simulink subsystem "celestialBodies"  (R2023b)
settings: Solver=VariableStepAuto  StartTime=0.0  StopTime=10.0  RelTol=1e-3
undefined symbols (not defined in the file or in its folder): Environment, phi, phi_dot, psi, psi_dot, theta, theta_dot
libraries: dyn_lib x2
settings Model: DataDictionary=Scenario.sldd  EnableAccessToBaseWorkspace=off  Creator=brent  LastModifiedBy=brent

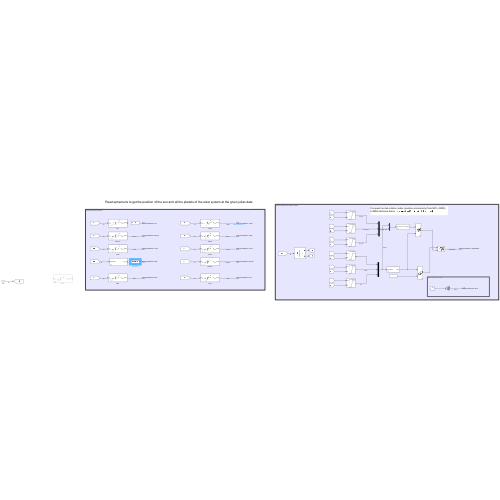
[thumbnail: Simulink's stored preview of the top-level diagram]
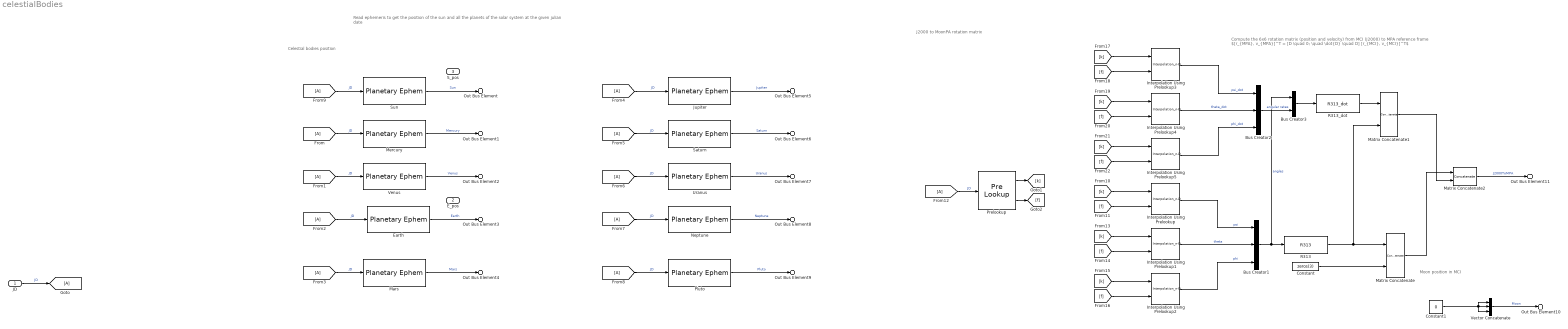
== system celestialBodies ==
  note: Compute the 6x6 rotation matrix (position and velocity) from MCI (J2000) to MPA reference frame $[r_{MPA}, v_{MPA}]^T = [D \quad 0; \quad \dot{D} \quad D] [r_{MCI}, v_{MCI}]^T$
  note: Read ephemeris to get the position of the sun and all the planets of the solar system at the given julian date
  note: Moon position in MCI
  note: J2000 to MoonPA rotation matrix
  note: Celestial bodies position
  JD : Inport
  E_pos : Inport  Port=2
  S_pos : Inport  Port=3
  Bus Creator1 : BusCreator  Inputs=psi,theta,phi
  Bus Creator2 : BusCreator  Inputs=psi_dot,theta_dot,phi_dot
  Bus Creator3 : BusCreator  Inputs=2
  Constant : Constant  Value=zeros(3)
  Constant1 : Constant  Value=0
  Earth : PlanetaryEphem  ephemerisModel=DE421  center=Moon  target=Earth  outputVelocity=off
  From{,1..9,12} (11 alike) : From
  Goto : Goto
  Interpolation Using Prelookup : Interpolation_n-D  NumberOfTableDimensions=1  Table=Environment.Moon.orientation.value(:,1)  InternalRulePriority=Speed
      settings: InputPortMap=u0,u1
  Interpolation Using Prelookup1 : Interpolation_n-D  NumberOfTableDimensions=1  Table=Environment.Moon.orientation.value(:,2)  InternalRulePriority=Speed
      settings: InputPortMap=u0,u1
  Interpolation Using Prelookup2 : Interpolation_n-D  NumberOfTableDimensions=1  Table=Environment.Moon.orientation.value(:,3)  InternalRulePriority=Speed
      settings: InputPortMap=u0,u1
  Interpolation Using Prelookup3 : Interpolation_n-D  NumberOfTableDimensions=1  Table=Environment.Moon.orientation_dot.value(:,1)  InternalRulePriority=Speed
      settings: InputPortMap=u0,u1
  Interpolation Using Prelookup4 : Interpolation_n-D  NumberOfTableDimensions=1  Table=Environment.Moon.orientation_dot.value(:,2)  InternalRulePriority=Speed
      settings: InputPortMap=u0,u1
  Interpolation Using Prelookup5 : Interpolation_n-D  NumberOfTableDimensions=1  Table=Environment.Moon.orientation_dot.value(:,3)  InternalRulePriority=Speed
      settings: InputPortMap=u0,u1
  Jupiter : PlanetaryEphem  ephemerisModel=DE421  center=Moon  target=Jupiter  outputVelocity=off
  Mars : PlanetaryEphem  ephemerisModel=DE421  center=Moon  target=Mars  outputVelocity=off
  Matrix Concatenate : Concatenate  Mode=Multidimensional array  ConcatenateDimension=2
  Matrix Concatenate1 : Concatenate  Mode=Multidimensional array  ConcatenateDimension=2
  Matrix Concatenate2 : Concatenate  Mode=Multidimensional array
  Mercury : PlanetaryEphem  ephemerisModel=DE421  center=Moon  target=Mercury  outputVelocity=off
  Neptune : PlanetaryEphem  ephemerisModel=DE421  center=Moon  target=Neptune  outputVelocity=off
  Pluto : PlanetaryEphem  ephemerisModel=DE421  center=Moon  target=Pluto  outputVelocity=off
  Prelookup : PreLookup  BreakpointsData=Environment.Moon.jd_interval.value  BeginIndexSearchUsingPreviousIndexResult=on  ExtrapMethod=Linear
  R313 : dyn_lib/R313
      settings: SourceProductName=Dynamics library
  R313_dot : dyn_lib/R313_dot
      settings: SourceProductName=Dynamics library
  Saturn : PlanetaryEphem  ephemerisModel=DE421  center=Moon  target=Saturn  outputVelocity=off
  "Sun " : PlanetaryEphem  ephemerisModel=DE421  center=Moon  target=Sun  outputVelocity=off
  Uranus : PlanetaryEphem  ephemerisModel=DE421  center=Moon  target=Uranus  outputVelocity=off
  Vector Concatenate : Concatenate  NumInputs=3
  Venus : PlanetaryEphem  ephemerisModel=DE421  center=Moon  target=Venus  outputVelocity=off
  Out Bus Element : Outport  PortName=celestialBodies  Element=Sun
  Out Bus Element1 : Outport  PortName=celestialBodies  Element=Mercury
  Out Bus Element2 : Outport  PortName=celestialBodies  Element=Venus
  Out Bus Element3 : Outport  PortName=celestialBodies  Element=Earth
  Out Bus Element4 : Outport  PortName=celestialBodies  Element=Mars
  Out Bus Element5 : Outport  PortName=celestialBodies  Element=Jupiter
  Out Bus Element6 : Outport  PortName=celestialBodies  Element=Saturn
  Out Bus Element7 : Outport  PortName=celestialBodies  Element=Uranus
  Out Bus Element8 : Outport  PortName=celestialBodies  Element=Neptune
  Out Bus Element9 : Outport  PortName=celestialBodies  Element=Pluto
  Out Bus Element10 : Outport  PortName=celestialBodies  Element=Moon
  Out Bus Element11 : Outport  PortName=celestialBodies  Element=J2000ToMPA
  wires:
  From/1 -> Mercury/1  "JD"
  From1/1 -> Venus/1  "JD"
  From3/1 -> Mars/1  "JD"
  From6/1 -> Uranus/1  "JD"
  From4/1 -> Jupiter/1  "JD"
  From5/1 -> Saturn/1  "JD"
  From7/1 -> Neptune/1  "JD"
  From8/1 -> Pluto/1  "JD"
  From9/1 -> "Sun "/1  "JD"
  Mercury/1 -> Out Bus Element1/1  "Mercury"
  Venus/1 -> Out Bus Element2/1  "Venus"
  Mars/1 -> Out Bus Element4/1  "Mars"
  Jupiter/1 -> Out Bus Element5/1  "Jupiter"
  Saturn/1 -> Out Bus Element6/1  "Saturn"
  Uranus/1 -> Out Bus Element7/1  "Uranus"
  Neptune/1 -> Out Bus Element8/1  "Neptune"
  Pluto/1 -> Out Bus Element9/1  "Pluto"
  JD/1 -> Goto/1  "JD"
  Prelookup/1 -> [k]
  Prelookup/2 -> [f]
  From12/1 -> Prelookup/1  "JD"
  [k] -> Interpolation Using Prelookup/1
  [f] -> Interpolation Using Prelookup/2
  [f] -> Interpolation Using Prelookup1/2
  [k] -> Interpolation Using Prelookup1/1
  [f] -> Interpolation Using Prelookup2/2
  [k] -> Interpolation Using Prelookup2/1
  [f] -> Interpolation Using Prelookup3/2
  [k] -> Interpolation Using Prelookup3/1
  [f] -> Interpolation Using Prelookup4/2
  [k] -> Interpolation Using Prelookup4/1
  [f] -> Interpolation Using Prelookup5/2
  [k] -> Interpolation Using Prelookup5/1
  Interpolation Using Prelookup1/1 -> Bus Creator1/2  "theta"
  Bus Creator1/1 -> R313/1, Bus Creator3/1  "angles"
  Interpolation Using Prelookup3/1 -> Bus Creator2/1  "psi_dot"
  Interpolation Using Prelookup4/1 -> Bus Creator2/2  "theta_dot"
  Interpolation Using Prelookup5/1 -> Bus Creator2/3  "phi_dot"
  Bus Creator2/1 -> Bus Creator3/2  "angular rates"
  Constant/1 -> Matrix Concatenate/2
  R313_dot/1 -> Matrix Concatenate1/1
  Bus Creator3/1 -> R313_dot/1
  Matrix Concatenate/1 -> Matrix Concatenate2/1
  Matrix Concatenate1/1 -> Matrix Concatenate2/2
  Interpolation Using Prelookup/1 -> Bus Creator1/1  "psi"
  Interpolation Using Prelookup2/1 -> Bus Creator1/3  "phi"
  Constant1/1 -> Vector Concatenate/2, Vector Concatenate/3, Vector Concatenate/1
  Matrix Concatenate2/1 -> Out Bus Element11/1  "J2000ToMPA"
  Vector Concatenate/1 -> Out Bus Element10/1  "Moon"
  R313/1 -> Matrix Concatenate/1, Matrix Concatenate1/2
  From2/1 -> Earth/1  "JD"
  Earth/1 -> Out Bus Element3/1  "Earth"
  "Sun "/1 -> Out Bus Element/1  "Sun"
